simulink model "separate"  (R2015b)
settings: Solver=VariableStepAuto  StartTime=0.0  StopTime=200  RelTol=1e-3
values from neighbouring files (symbols this model uses):
  alpha_const = 0.0    (= 0)    [averagedRelayOutput.m]    (also in bursting_linearised.m = 0.1; fastSlow.m; manParamsNullclines.m; manipulateParameters.m = getappdata(hObject.Parent,'alpha_const'))
  beta = 0.37    [averagedRelayOutput.m]    (also in bursting_linearised.m = 0.27; compareApproximations.m = 1.5; fastSlow.m; fast_nullcline_winged_cusp.m = 0.5)
  gamma = 0    [averagedRelayOutput.m]    (also in bursting_linearised.m = 1; compareApproximations.m = 1; fastSlow.m; fast_nullcline_winged_cusp.m = 1)
  kb = -0.5    [averagedRelayOutput.m]    (also in fastSlow.m; findPeriodForAsymmOscill.m = 0.5; originalModel2.m; product.m)
  ts = 1    [averagedRelayOutput.m]    (also in bursting_linearised.m; compareApproximations.m; fastSlow.m; fast_nullcline_winged_cusp.m)
  tus = 800    [averagedRelayOutput.m]    (also in bursting_linearised.m; fastSlow.m; manParamsNullclines.m; manipulateParameters.m = getappdata(hObject.Parent,'tus'))
  ultra_slow_plant_X0 = 0.45    [averagedRelayOutput.m]    (also in bursting_linearised.m = 0; fastSlow.m; hRose.m = 2000; manParamsNullclines.m)
settings Model: Creator=rajiv  LastModifiedBy=rajiv

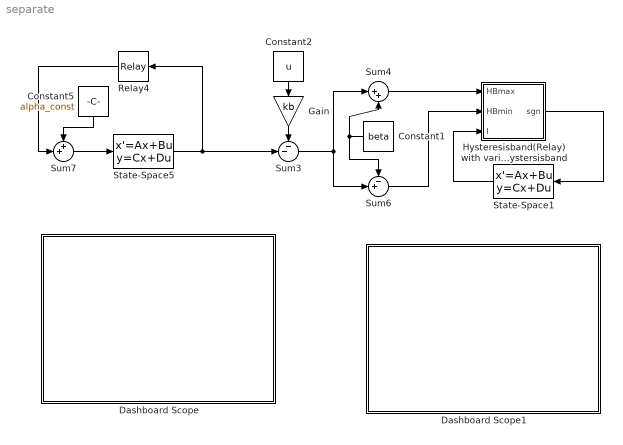
== system separate ==
  Constant1 : Constant  Value=beta
  Constant2 : Constant  Value=u
  Constant5 : Constant  Value=alpha_const
  Dashboard Scope : Subsystem  DialogController=hmiCreateDDGDialog  IsWebBlock=on  mask(MWDashboardBlock){webBlockId=0715e74d-8397-4baf-8bea-cbae6d72404b, webBlockType=sdiscope, ShowInitialText=on, HMISrcModelName=separate}
      mask prompts: webBlockId "WebBlock Id"; webBlockType "WebBlock Type"; HMISrcModelName "Source Model"
      mask Help: helpview([docroot '/mapfiles/simulink.map'], 'hmi_scope')
      mask Display:
      | if strcmp(get_param(bdroot(gcb),'BlockDiagramType'), 'library')
      |     image([(matlabroot) '/toolbox/simulink/hmi/icons/DashboardScope.png']);
      | end
  Dashboard Scope1 : Subsystem  DialogController=hmiCreateDDGDialog  IsWebBlock=on  mask(MWDashboardBlock){webBlockId=0f46d1a0-6c93-4c8b-92e7-dc79eecd858f, webBlockType=sdiscope, ShowInitialText=on, HMISrcModelName=separate}
      mask prompts: webBlockId "WebBlock Id"; webBlockType "WebBlock Type"; HMISrcModelName "Source Model"
      mask Help: helpview([docroot '/mapfiles/simulink.map'], 'hmi_scope')
      mask Display:
      | if strcmp(get_param(bdroot(gcb),'BlockDiagramType'), 'library')
      |     image([(matlabroot) '/toolbox/simulink/hmi/icons/DashboardScope.png']);
      | end
  Gain : Gain  Gain=kb
  Hysteresisband(Relay)with variable hystersisband : MATLAB Function  TreatAsAtomicUnit=on
  Relay4 : Relay  OnSwitchValue=beta-0.5*(u-1/ts-0.5*gamma)  OffSwitchValue=beta  OnOutputValue=0.2  OffOutputValue=-1
  State-Space1 : StateSpace  A=-1/ts  B=1/ts  D=0.5*1*gamma  X0=0
  State-Space5 : StateSpace  A=-1/tus  B=-1/tus  D=0  X0=ultra_slow_plant_X0
  Sum3 : Sum  Inputs=--|
  Sum4 : Sum  Inputs=|++
  Sum6 : Sum  Inputs=-+|
  Sum7 : Sum  Inputs=++|
  wires:
  Constant5/1 -> Sum7/1
  Sum7/1 -> State-Space5/1
  Relay4/1 -> Sum7/2
  State-Space5/1 -> Sum3/2, Relay4/1
  Hysteresisband(Relay)with variable hystersisband/1(sgn) -> State-Space1/1
  State-Space1/1 -> Hysteresisband(Relay)with variable hystersisband/3(I)
  Constant2/1 -> Gain/1
  Gain/1 -> Sum3/1
  Sum3/1 -> Sum4/1, Sum6/2
  Sum4/1 -> Hysteresisband(Relay)with variable hystersisband/1(HBmax)
  Constant1/1 -> Sum6/1, Sum4/2
  Sum6/1 -> Hysteresisband(Relay)with variable hystersisband/2(HBmin)

== system separate/Dashboard Scope ==

== system separate/Dashboard Scope1 ==

== matlab function separate/Hysteresisband(Relay)with variable hystersisband ==
  data: HBmax input; sgn output; HBmin input; I input
function sgn  = fcn(HBmax,HBmin,I)

%#codegen
if (HBmax>I)&&(I>HBmin)
     sgn=1;
else
     sgn=-1;
end
